simulink model "shiyan4_1"  (R2023a)
settings: Solver=VariableStepAuto  StartTime=0.0  StopTime=20  RelTol=1e-3
settings Model: Creator=VICTOR7  LastModifiedBy=VICTOR7

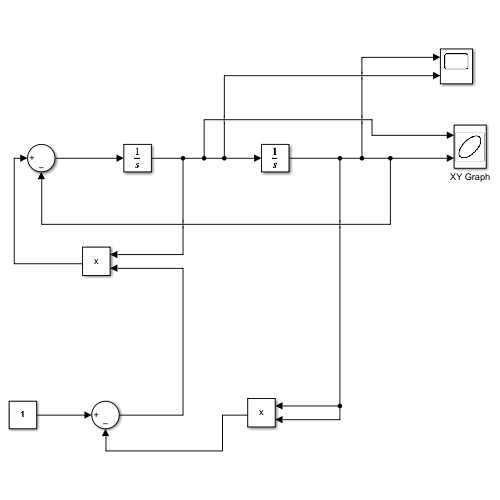
[thumbnail: Simulink's stored preview of the top-level diagram]
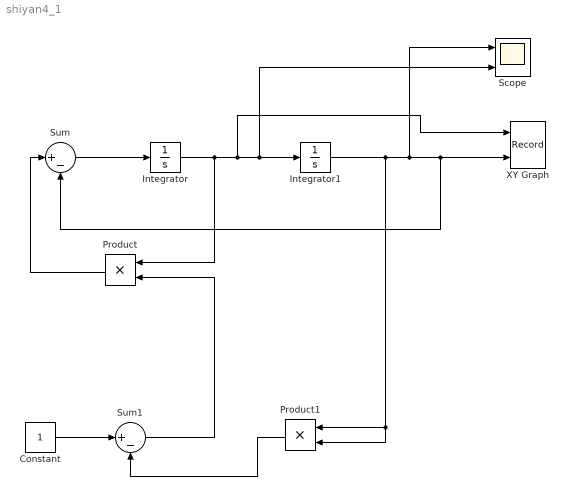
== system shiyan4_1 ==
  Constant : Constant
  Integrator : Integrator
  Integrator1 : Integrator  InitialCondition=1
  Product : Product
  Product1 : Product
  Scope : Scope  NumInputPorts=2
  Sum : Sum  Inputs=|+-
  Sum1 : Sum  Inputs=|+-
  XY Graph : Record  FileSettingsInternal="{\"entries\":[{\"content\":{\"excelSettings\":{\"content\":{},\"type\":\"Streamout.ExcelSettings\"}},\"type\":\"Streamout.FileSettingStorage\",\"uuid\":\"8c1716bc-0c24-44b1-9262-a57f2700d98a\"}],\"packageUris\":[\"http://schema.mathworks.com/mf0/streamout_blocks/R2020a\"],\"version\":\"1.0\"}"  Layout=[1 1]  SignalsInternal="{\"entries\":[{\"content\":{\"signals\":[{\"content\":{\"blockPath\":[\"untitled/XY Graph\"],\"dimensions\":[1],\"domain\":\"untitled/XY Graph\",\"lineColor\":\"#a2142f\",\"plots\":[1],\"port\":1,\"sid\":[\"\"],\"signalID\":194,\"signalName\":\"Integrator\"},\"type\":\"RecordBlkView.Signal\",\"uuid\":\"7013b3f7-f4ab-4e6e-b95c-a2f43c0033f1\"},{\"content\":{\"blockPath\":[\"untitled/XY Graph\"],\"dimensions\":[1],\"domain\":\"untitled/XY Graph\",\"lineColor\":\"#139fff\",\"plots\":[1],\"port\":2,\"sid\":[\"\"],\"signalID\":198,\"signalName\":\"Integrator1\"},\"type\":\"RecordBlkView.Signal\",\"uuid\":\"e71c923c-b8fa-4d00-8e61-e78550c3d4dd\"}]},\"type\":\"RecordBlkView.InputSignals\",\"uuid\":\"38ca1585-f7ae-429f-90fb-b397e3adb104\"}],\"packageUris\":[\"http://schema.mathworks.com/mf0/streamout_blocks/R2020a\"],\"version\":\"1.0\"}"  VisualizationBindings="{\"xyplotplugin\":{\"info\":[{\"series\":[{\"bindingParametersList\":[{\"parameter\":\"X-Axis\",\"signalID\":194,\"signalName\":\"Integrator\"},{\"parameter\":\"Y-Axis\",\"signalID\":198,\"signalName\":\"Integrator1\"}],\"seriesID\":25969}],\"subplotID\":1}]}}"  CompatibilityTag=XY
  wires:
  Integrator/1 -> Product/1, XY Graph/1, Integrator1/1, Scope/2
  Sum/1 -> Integrator/1
  Constant/1 -> Sum1/1
  Product/1 -> Sum/1
  Sum1/1 -> Product/2
  Product1/1 -> Sum1/2
  Integrator1/1 -> Product1/2, Product1/1, Scope/1, XY Graph/2, Sum/2
